simulink library "srx_platform"  (Simulink 8.2)
settings: Solver=ode1  StartTime=0.0  StopTime=Inf  FixedStep=0.001  RelTol=1e-3
PostLoadFcn:
  | , if any(exist('dsrtsu_mdlpostloadfcn', 'file') == [2, 3, 6]), try dsrtsu_mdlpostloadfcn('Execute', bdroot); catch fprintf('Error in PostLoadFcn (dsrtsu_mdlpostloadfcn) for model "%s":\n %s\n', bdroot, lasterr); end, end,
libraries: rtican x23, rtiethernetudplib x4, srx_initialize x4, rtiflashlib x2, topr5_adapter x1
(part 6 of 6)

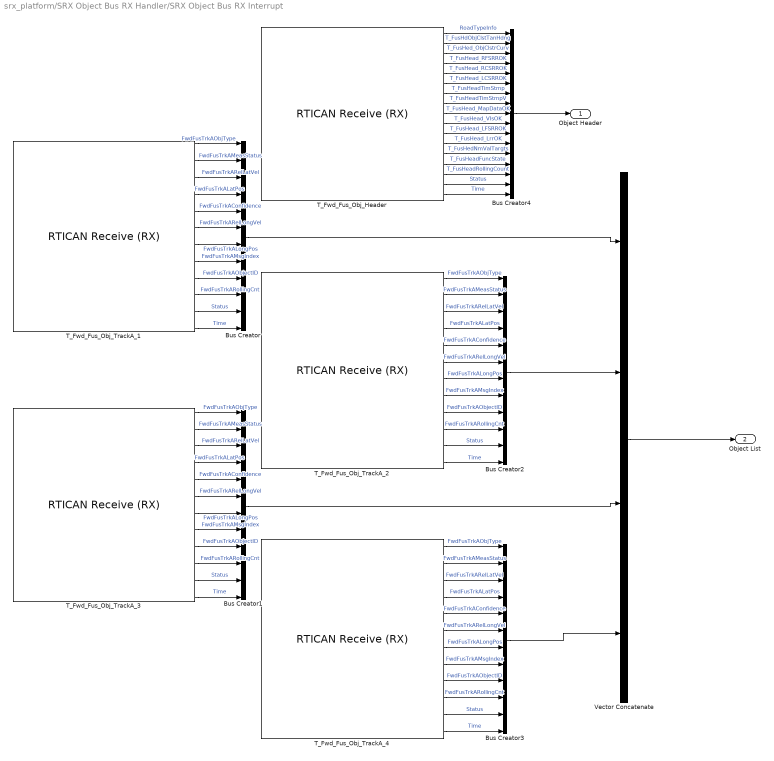
== system srx_platform/SRX Object Bus RX Handler/SRX Object Bus RX Interrupt ==
  Bus Creator{,1..3} (4 alike) : BusCreator  Inputs='FwdFusTrkAObjType','FwdFusTrkAMeasStatus','FwdFusTrkARelLatVel','FwdFusTrkALatPos','FwdFusTrkAConfidence','FwdFusTrkARelLongVel','FwdFusTrkALongPos','FwdFusTrkAMsgIndex','FwdFusTrkAObjectID','FwdFusTrkARollingCnt','Status','Time'  OutDataTypeStr=Bus: FusObjectTrackA  NonVirtualBus=on
  Bus Creator4 : BusCreator  Inputs=17
  T_Fwd_Fus_Obj_Header : rtican/RTICAN Receive (RX)   Reserved1=[]  Reserved2=[]  Reserved3=[]  Reserved4=[]  SfcnMessage=[]  Msg_Struct=[]  BoardTypeNo=[]  BoardNo=[]  ChannelNo=[]  Parameters=[]  DialogFcn=[]  UnitName=[]  Revision=[]  UnitValues=[]  DSProperties=struct('RTI',struct('Version',uint32(5),'BlockType',struct('isSLSource',uint8(1),'isSLSink',uint8(1),'isHWSource',uint8(0),'isHWSink',uint8(0),'isSetup',uint8(0),'isInline',uint8(1),'isNonInline',uint8(0),'isInterrupt',uint8(0),'isChannelwise',uint8(0)),'IOBoardType','RTICAN','UnitType','MESSAGE','Identifier','RX','DialogType','MSVC','BlockSet','RTICAN','SlaveProcessor','CAN'))  RTIBlockInterface=struct('OutputPortsWidth',int32([1 1 1 1 1 1 1 1 1 1 1 1 1 1 1 1 1]),'OutputPortsActive',[1 1 1 1 1 1 1 1 1 1 1 1 1 1 1 1 1],'OutputPortsName',{{'RoadTypeInfo','T_FusHdObjClstTanHdng','T_FusHed_ObjClstrCurv','T_FusHead_RFSRROK','T_FusHead_RCSRROK','T_FusHead_LCSRROK','T_FusHeadTimStmp','T_FusHeadTimStmpV','T_FusHead_MapDataOK','T_FusHead_VIsOK','T_FusHead_LFSRROK','T_FusHead_LrrOK','T_FusHedNmValTargts','T_FusHeadFuncState','T_FusHeadRollingCount',['RX status'],['RX time']}},'OutputPortsDataType',{{'SS_DOUBLE','SS_DOUBLE','SS_DOUBLE','SS_DOUBLE','SS_DOUBLE','SS_DOUBLE','SS_DOUBLE','SS_DOUBLE','SS_DOUBLE','SS_DOUBLE','SS_DOUBLE','SS_DOUBLE','SS_DOUBLE','SS_DOUBLE','SS_DOUBLE','SS_DOUBLE','SS_DOUBLE'}},'OutputPortsLabel',{{'RoadTypeInfo','T_FusHdObjClstTanHdng','T_FusHed_ObjClstrCurv','T_FusHead_RFSRROK','T_FusHead_RCSRROK','T_FusHead_LCSRROK','T_FusHeadTimStmp','T_FusHeadTimStmpV','T_FusHead_MapDataOK','T_FusHead_VIsOK','T_FusHead_LFSRROK','T_FusHead_LrrOK','T_FusHedNmValTargts','T_FusHeadFuncState','T_FusHeadRollingCount','',''}},'OutputPortsLabelMode','ON','InputPortsWidth',int32(0),'InputPortsActive',0,'DialogFcn','rtican_message_interface_gui','BlockDisplay',{{'','center'}},'IconTransparency','on','ParameterTunableNames',{{}},'InitLevel',3,'BlockName',struct('Token',{{'T_Fwd_Fus_Obj_Header'}}),'SampleTime',{{-1}},'TriggerPort',{{'none'}},'EnablePort',{{'none'}})  RTIBlockParameters=struct('BoardTypeNo',{{1,'OFF',[]}},'BoardNo',{{1,'ON',[1 16]}},'ChannelNo',{{2,'ON',[1 2]}},'Parameters',{{struct('DataFileSupport',struct('DataFileSelectedMaster',1,'DataFileSelectedLocal',0,'DataFileName','c:\users\leidos\development\carmaplatform\microautobox\src\data_files\globala_fo.dbc|','DataFileDate',{{{['23-Jul-2015 14:24:26']}}},'SelectedFile',['<no file selected>']),'Options',struct('StatusSelected',1,'TimeSelected',1,'DeltaTimeSelected',0,'BytePortSelected',0,'MessageLengthSelected',0,'TriggerPort',struct('Selected',0,'TriggerType',0),'UserCoding',struct('Selected',0,'InterfaceFile','UserDecodingFile','FcnName','UserDecodeFcn','InportSelected',0,'InportWidth',1,'OutportSelected',0,'OutportWidth',1),'EnablePortSelected',0,'SignalOnPortnameSelected',1,'UseRXService',1),'Message',struct('MsgOnBlocknameSelected',1,'MsgName','T_Fwd_Fus_Obj_Header','MsgIdFormat',0,'MsgId',1808,'MsgLength',7,'NumSignals',15,'SampleTime',-1,'Signal',struct('SgnName',{'RoadTypeInfo','T_FusHdObjClstTanHdng','T_FusHed_ObjClstrCurv','T_FusHead_RFSRROK','T_FusHead_RCSRROK','T_FusHead_LCSRROK','T_FusHeadTimStmp','T_FusHeadTimStmpV','T_FusHead_MapDataOK','T_FusHead_VIsOK','T_FusHead_LFSRROK','T_FusHead_LrrOK','T_FusHedNmValTargts','T_FusHeadFuncState','T_FusHeadRollingCount'},'SgnStartBit',{5,8,16,29,30,31,32,43,44,45,46,47,48,52,54},'SgnLength',{3,8,13,1,1,1,11,1,1,1,1,1,4,2,2},'SgnType',{0,0,0,0,0,0,0,0,0,0,0,0,0,0,0},'ModeValue',{-1,-1,-1,-1,-1,-1,-1,-1,-1,-1,-1,-1,-1,-1,-1},'DataType',{0,1,1,0,0,0,0,0,0,0,0,0,0,0,0},'ByteLayout',{2,2,2,2,2,2,2,2,2,2,2,2,2,2,2},'Factor',{1,0.002,5e-05,1,1,1,1,1,1,1,1,1,1,1,1},'Offset',{0,0,0,0,0,0,0,0,0,0,0,0,0,0,0},'SgnComment',{{''},{''},{''},{''},{''},{''},{''},{''},{''},{''},{''},{''},{''},{''},{''}},'SgnUnit',{'','m/m','1/m','','','','ms','','','','','','','',''},'Min',{0,-0.256,-0.2048,0,0,0,0,0,0,0,0,0,0,0,0},'Max',{7,0.254,0.20475,1,1,1,2047,1,1,1,1,1,15,3,3},'SLDataType',{'SS_DOUBLE','SS_DOUBLE','SS_DOUBLE','SS_DOUBLE','SS_DOUBLE','SS_DOUBLE','SS_DOUBLE','SS_DOUBLE','SS_DOUBLE','SS_DOUBLE','SS_DOUBLE','SS_DOUBLE','SS_DOUBLE','SS_DOUBLE','SS_DOUBLE'}),'MsgIdNumFormat',1,'MsgComment',{{''}}),'Version',1.2,'general',struct('isFromLib',0)),'OFF',[]}},'GroupId',{{struct('Group',{{'RTICAN'}},'No',2,'Behavior',{{'NAMECHANGE'}},'BlockType',{{'SINK'}},'NameChangeFlag',0),'OFF',[]}},'SFcnRTICANMessage',{{struct('MsgType','RX','SFcnPortType','Scalar','MsgName','T_Fwd_Fus_Obj_Header','MsgIdFormat','STD','MsgId',1808,'MsgLength',7,'NumSignals',15,'SampleTime',-1,'Signal',struct('SgnName',{'RoadTypeInfo','T_FusHdObjClstTanHdng','T_FusHed_ObjClstrCurv','T_FusHead_RFSRROK','T_FusHead_RCSRROK','T_FusHead_LCSRROK','T_FusHeadTimStmp','T_FusHeadTimStmpV','T_FusHead_MapDataOK','T_FusHead_VIsOK','T_FusHead_LFSRROK','T_FusHead_LrrOK','T_FusHedNmValTargts','T_FusHeadFuncState','T_FusHeadRollingCount'},'SgnStartBit',{5,8,16,29,30,31,32,43,44,45,46,47,48,52,54},'SgnLength',{3,8,13,1,1,1,11,1,1,1,1,1,4,2,2},'SgnType',{'standard','standard','standard','standard','standard','standard','standard','standard','standard','standard','standard','standard','standard','standard','standard'},'ModeValue',{-1,-1,-1,-1,-1,-1,-1,-1,-1,-1,-1,-1,-1,-1,-1},'DataType',{['unsigned int'],['signed int'],['signed int'],['unsigned int'],['unsigned int'],['unsigned int'],['unsigned int'],['unsigned int'],['unsigned int'],['unsigned int'],['unsigned int'],['unsigned int'],['unsigned int'],['unsigned int'],['unsigned int']},'ByteLayout',{['motorola back.'],['motorola back.'],['motorola back.'],['motorola back.'],['motorola back.'],['motorola back.'],['motorola back.'],['motorola back.'],['motorola back.'],['motorola back.'],['motorola back.'],['motorola back.'],['motorola back.'],['motorola back.'],['motorola back.']},'Factor',{1,0.002,5e-05,1,1,1,1,1,1,1,1,1,1,1,1},'Offset',{0,0,0,0,0,0,0,0,0,0,0,0,0,0,0},'SLDataType',{'SS_DOUBLE','SS_DOUBLE','SS_DOUBLE','SS_DOUBLE','SS_DOUBLE','SS_DOUBLE','SS_DOUBLE','SS_DOUBLE','SS_DOUBLE','SS_DOUBLE','SS_DOUBLE','SS_DOUBLE','SS_DOUBLE','SS_DOUBLE','SS_DOUBLE'}),'StatusSelected','yes','TimeSelected','yes','DeltaTimeSelected','no','BytePortSelected','no','MessageLengthSelected','no','TriggerPort',struct('Selected','no','TriggerType',0),'UserCoding',struct('Selected','no','InterfaceFile','UserDecodingFile','FcnName','UserDecodeFcn','InportSelected','no','InportWidth',1,'OutportSelected','no','OutportWidth',1),'EnablePortSelected','no','UseRXService','yes','BoardType','DS1','BoardNo',1,'ControllerNo',2),'OFF',[]}},'TLCFileName',{{'rtican_rx_message','OFF',[]}})  RTISFcnParameters=struct('SFcnRTICANMessage','struct','TLCFileName','char')  RTIBlockParaDefault=struct('BoardTypeNo',4302,'BoardNo',1,'ChannelNo',1,'Parameters',struct('DataFileSupport',struct('DataFileSelectedMaster',0,'DataFileSelectedLocal',0,'DataFileName','','DataFileDate','','SelectedFile',['<no file selected>']),'Options',struct('StatusSelected',1,'TimeSelected',1,'DeltaTimeSelected',1,'BytePortSelected',0,'MessageLengthSelected',0,'TriggerPort',struct('Selected',0,'TriggerType','rising'),'UserCoding',struct('Selected',0,'InterfaceFile','UserDecodingFile','FcnName','UserDecodeFcn','InportSelected',0,'InportWidth',1,'OutportSelected',0,'OutportWidth',1),'EnablePortSelected',0,'SignalOnPortnameSelected',1,'UseRXService',0),'Message',struct('MsgOnBlocknameSelected',0,'MsgName',['RX Message'],'MsgIdFormat',0,'MsgId',100,'MsgLength',8,'NumSignals',1,'SampleTime',-1,'Signal',struct('SgnName',['RX signal'],'SgnStartBit',0,'SgnLength',8,'SgnType',0,'ModeValue',-1,'DataType',0,'SLDataType','SS_DOUBLE','ByteLayout',0,'Factor',1,'Offset',0,'Min',0,'Max',255,'SgnComment',{{}},'SgnUnit',''),'MsgIdNumFormat',0,'MsgComment',{{''}}),'Version',1.2,'general',struct('isFromLib',1)),'GroupId',struct('Group',{{'RTICAN'}},'No',1,'Behavior',{{'NAMECHANGE'}},'BlockType',{{'SINK'}},'NameChangeFlag',0),'SFcnRTICANMessage',struct('MsgType','RX','MsgName',['RX Message'],'MsgIdFormat','STD','MsgId',100,'MsgLength',8,'NumSignals',1,'SampleTime',-1,'Signal',struct('SgnName',['RX signal'],'SgnStartBit',0,'SgnLength',8,'SgnType','standard','ModeValue',-1,'DataType',['unsigned int'],'ByteLayout',['little endian'],'SLDataType','SS_DOUBLE','Factor',1,'Offset',0),'StatusSelected','yes','TimeSelected','yes','DeltaTimeSelected','yes','BytePortSelected','no','MessageLengthSelected','no','EnablePortSelected','no','UserCoding',struct('Selected','no','InterfaceFile','UserDecodingFile','FcnName','UserDecodeFcn','InportSelected','no','InportWidth',1,'OutportSelected','no','OutportWidth',1),'TriggerPort',struct('Selected','no','TriggerType','rising'),'UseRXService','no','BoardType','DS4302','BoardNo',1,'ControllerNo',1,'SFcnPortType','Scalar'),'TLCFileName','rtican_rx_message')
      settings: AttributesFormatString=Group Id: RTICAN2\n
  T_Fwd_Fus_Obj_TrackA_1 : rtican/RTICAN Receive (RX)   Reserved1=[]  Reserved2=[]  Reserved3=[]  Reserved4=[]  SfcnMessage=[]  Msg_Struct=[]  BoardTypeNo=[]  BoardNo=[]  ChannelNo=[]  Parameters=[]  DialogFcn=[]  UnitName=[]  Revision=[]  UnitValues=[]  DSProperties=struct('RTI',struct('Version',uint32(5),'BlockType',struct('isSLSource',uint8(1),'isSLSink',uint8(1),'isHWSource',uint8(0),'isHWSink',uint8(0),'isSetup',uint8(0),'isInline',uint8(1),'isNonInline',uint8(0),'isInterrupt',uint8(0),'isChannelwise',uint8(0)),'IOBoardType','RTICAN','UnitType','MESSAGE','Identifier','RX','DialogType','MSVC','BlockSet','RTICAN','SlaveProcessor','CAN'))  RTIBlockInterface=struct('OutputPortsWidth',int32([1 1 1 1 1 1 1 1 1 1 1 1]),'OutputPortsActive',[1 1 1 1 1 1 1 1 1 1 1 1],'OutputPortsName',{{'FwdFusTrkAObjType','FwdFusTrkAMeasStatus','FwdFusTrkARelLatVel','FwdFusTrkALatPos','FwdFusTrkAConfidence','FwdFusTrkARelLongVel','FwdFusTrkALongPos','FwdFusTrkAMsgIndex','FwdFusTrkAObjectID','FwdFusTrkARollingCnt',['RX status'],['RX time']}},'OutputPortsDataType',{{'SS_DOUBLE','SS_DOUBLE','SS_DOUBLE','SS_DOUBLE','SS_DOUBLE','SS_DOUBLE','SS_DOUBLE','SS_DOUBLE','SS_DOUBLE','SS_DOUBLE','SS_DOUBLE','SS_DOUBLE'}},'OutputPortsLabel',{{'FwdFusTrkAObjType','FwdFusTrkAMeasStatus','FwdFusTrkARelLatVel','FwdFusTrkALatPos','FwdFusTrkAConfidence','FwdFusTrkARelLongVel','FwdFusTrkALongPos','FwdFusTrkAMsgIndex','FwdFusTrkAObjectID','FwdFusTrkARollingCnt','',''}},'OutputPortsLabelMode','ON','InputPortsWidth',int32(0),'InputPortsActive',0,'DialogFcn','rtican_message_interface_gui','BlockDisplay',{{'','center'}},'IconTransparency','on','ParameterTunableNames',{{}},'InitLevel',3,'BlockName',struct('Token',{{'T_Fwd_Fus_Obj_TrackA_1'}}),'SampleTime',{{-1}},'TriggerPort',{{'none'}},'EnablePort',{{'none'}})  RTIBlockParameters=struct('BoardTypeNo',{{1,'OFF',[]}},'BoardNo',{{1,'ON',[1 16]}},'ChannelNo',{{2,'ON',[1 2]}},'Parameters',{{struct('DataFileSupport',struct('DataFileSelectedMaster',1,'DataFileSelectedLocal',0,'DataFileName','c:\users\leidos\development\carmaplatform\microautobox\src\data_files\globala_fo.dbc|','DataFileDate',{{{['23-Jul-2015 14:24:26']}}},'SelectedFile',['<no file selected>']),'Options',struct('StatusSelected',1,'TimeSelected',1,'DeltaTimeSelected',0,'BytePortSelected',0,'MessageLengthSelected',0,'TriggerPort',struct('Selected',0,'TriggerType',0),'UserCoding',struct('Selected',0,'InterfaceFile','UserDecodingFile','FcnName','UserDecodeFcn','InportSelected',0,'InportWidth',1,'OutportSelected',0,'OutportWidth',1),'EnablePortSelected',0,'SignalOnPortnameSelected',1,'UseRXService',1),'Message',struct('MsgOnBlocknameSelected',1,'MsgName','T_Fwd_Fus_Obj_TrackA_1','MsgIdFormat',0,'MsgId',1809,'MsgLength',8,'NumSignals',10,'SampleTime',-1,'Signal',struct('SgnName',{'FwdFusTrkAObjType','FwdFusTrkAMeasStatus','FwdFusTrkARelLatVel','FwdFusTrkALatPos','FwdFusTrkAConfidence','FwdFusTrkARelLongVel','FwdFusTrkALongPos','FwdFusTrkAMsgIndex','FwdFusTrkAObjectID','FwdFusTrkARollingCnt'},'SgnStartBit',{0,3,5,16,27,29,40,52,56,62},'SgnLength',{3,2,11,11,2,11,12,4,6,2},'SgnType',{0,0,0,0,0,0,0,0,0,0},'ModeValue',{-1,-1,-1,-1,-1,-1,-1,-1,-1,-1},'DataType',{0,0,1,1,0,1,1,0,0,0},'ByteLayout',{2,2,2,2,2,2,2,2,2,2},'Factor',{1,1,0.125,0.125,1,0.125,0.125,1,1,1},'Offset',{0,0,0,0,0,0,0,0,0,0},'SgnComment',{{''},{''},{''},{''},{''},{''},{''},{''},{''},{''}},'SgnUnit',{'','','m/s','m','','m/s','m','','',''},'Min',{0,0,-128,-128,0,-128,-256,0,0,0},'Max',{7,3,127.875,127.875,3,127.875,255.875,15,63,3},'SLDataType',{'SS_DOUBLE','SS_DOUBLE','SS_DOUBLE','SS_DOUBLE','SS_DOUBLE','SS_DOUBLE','SS_DOUBLE','SS_DOUBLE','SS_DOUBLE','SS_DOUBLE'}),'MsgIdNumFormat',1,'MsgComment',{{''}}),'Version',1.2,'general',struct('isFromLib',0)),'OFF',[]}},'GroupId',{{struct('Group',{{'RTICAN'}},'No',2,'Behavior',{{'NAMECHANGE'}},'BlockType',{{'SINK'}},'NameChangeFlag',0),'OFF',[]}},'SFcnRTICANMessage',{{struct('MsgType','RX','SFcnPortType','Scalar','MsgName','T_Fwd_Fus_Obj_TrackA_1','MsgIdFormat','STD','MsgId',1809,'MsgLength',8,'NumSignals',10,'SampleTime',-1,'Signal',struct('SgnName',{'FwdFusTrkAObjType','FwdFusTrkAMeasStatus','FwdFusTrkARelLatVel','FwdFusTrkALatPos','FwdFusTrkAConfidence','FwdFusTrkARelLongVel','FwdFusTrkALongPos','FwdFusTrkAMsgIndex','FwdFusTrkAObjectID','FwdFusTrkARollingCnt'},'SgnStartBit',{0,3,5,16,27,29,40,52,56,62},'SgnLength',{3,2,11,11,2,11,12,4,6,2},'SgnType',{'standard','standard','standard','standard','standard','standard','standard','standard','standard','standard'},'ModeValue',{-1,-1,-1,-1,-1,-1,-1,-1,-1,-1},'DataType',{['unsigned int'],['unsigned int'],['signed int'],['signed int'],['unsigned int'],['signed int'],['signed int'],['unsigned int'],['unsigned int'],['unsigned int']},'ByteLayout',{['motorola back.'],['motorola back.'],['motorola back.'],['motorola back.'],['motorola back.'],['motorola back.'],['motorola back.'],['motorola back.'],['motorola back.'],['motorola back.']},'Factor',{1,1,0.125,0.125,1,0.125,0.125,1,1,1},'Offset',{0,0,0,0,0,0,0,0,0,0},'SLDataType',{'SS_DOUBLE','SS_DOUBLE','SS_DOUBLE','SS_DOUBLE','SS_DOUBLE','SS_DOUBLE','SS_DOUBLE','SS_DOUBLE','SS_DOUBLE','SS_DOUBLE'}),'StatusSelected','yes','TimeSelected','yes','DeltaTimeSelected','no','BytePortSelected','no','MessageLengthSelected','no','TriggerPort',struct('Selected','no','TriggerType',0),'UserCoding',struct('Selected','no','InterfaceFile','UserDecodingFile','FcnName','UserDecodeFcn','InportSelected','no','InportWidth',1,'OutportSelected','no','OutportWidth',1),'EnablePortSelected','no','UseRXService','yes','BoardType','DS1','BoardNo',1,'ControllerNo',2),'OFF',[]}},'TLCFileName',{{'rtican_rx_message','OFF',[]}})  RTISFcnParameters=struct('SFcnRTICANMessage','struct','TLCFileName','char')  RTIBlockParaDefault=struct('BoardTypeNo',4302,'BoardNo',1,'ChannelNo',1,'Parameters',struct('DataFileSupport',struct('DataFileSelectedMaster',0,'DataFileSelectedLocal',0,'DataFileName','','DataFileDate','','SelectedFile',['<no file selected>']),'Options',struct('StatusSelected',1,'TimeSelected',1,'DeltaTimeSelected',1,'BytePortSelected',0,'MessageLengthSelected',0,'TriggerPort',struct('Selected',0,'TriggerType','rising'),'UserCoding',struct('Selected',0,'InterfaceFile','UserDecodingFile','FcnName','UserDecodeFcn','InportSelected',0,'InportWidth',1,'OutportSelected',0,'OutportWidth',1),'EnablePortSelected',0,'SignalOnPortnameSelected',1,'UseRXService',0),'Message',struct('MsgOnBlocknameSelected',0,'MsgName',['RX Message'],'MsgIdFormat',0,'MsgId',100,'MsgLength',8,'NumSignals',1,'SampleTime',-1,'Signal',struct('SgnName',['RX signal'],'SgnStartBit',0,'SgnLength',8,'SgnType',0,'ModeValue',-1,'DataType',0,'SLDataType','SS_DOUBLE','ByteLayout',0,'Factor',1,'Offset',0,'Min',0,'Max',255,'SgnComment',{{}},'SgnUnit',''),'MsgIdNumFormat',0,'MsgComment',{{''}}),'Version',1.2,'general',struct('isFromLib',1)),'GroupId',struct('Group',{{'RTICAN'}},'No',1,'Behavior',{{'NAMECHANGE'}},'BlockType',{{'SINK'}},'NameChangeFlag',0),'SFcnRTICANMessage',struct('MsgType','RX','MsgName',['RX Message'],'MsgIdFormat','STD','MsgId',100,'MsgLength',8,'NumSignals',1,'SampleTime',-1,'Signal',struct('SgnName',['RX signal'],'SgnStartBit',0,'SgnLength',8,'SgnType','standard','ModeValue',-1,'DataType',['unsigned int'],'ByteLayout',['little endian'],'SLDataType','SS_DOUBLE','Factor',1,'Offset',0),'StatusSelected','yes','TimeSelected','yes','DeltaTimeSelected','yes','BytePortSelected','no','MessageLengthSelected','no','EnablePortSelected','no','UserCoding',struct('Selected','no','InterfaceFile','UserDecodingFile','FcnName','UserDecodeFcn','InportSelected','no','InportWidth',1,'OutportSelected','no','OutportWidth',1),'TriggerPort',struct('Selected','no','TriggerType','rising'),'UseRXService','no','BoardType','DS4302','BoardNo',1,'ControllerNo',1,'SFcnPortType','Scalar'),'TLCFileName','rtican_rx_message')
      settings: AttributesFormatString=Group Id: RTICAN2\n
  T_Fwd_Fus_Obj_TrackA_2 : rtican/RTICAN Receive (RX)   Reserved1=[]  Reserved2=[]  Reserved3=[]  Reserved4=[]  SfcnMessage=[]  Msg_Struct=[]  BoardTypeNo=[]  BoardNo=[]  ChannelNo=[]  Parameters=[]  DialogFcn=[]  UnitName=[]  Revision=[]  UnitValues=[]  DSProperties=struct('RTI',struct('Version',uint32(5),'BlockType',struct('isSLSource',uint8(1),'isSLSink',uint8(1),'isHWSource',uint8(0),'isHWSink',uint8(0),'isSetup',uint8(0),'isInline',uint8(1),'isNonInline',uint8(0),'isInterrupt',uint8(0),'isChannelwise',uint8(0)),'IOBoardType','RTICAN','UnitType','MESSAGE','Identifier','RX','DialogType','MSVC','BlockSet','RTICAN','SlaveProcessor','CAN'))  RTIBlockInterface=struct('OutputPortsWidth',int32([1 1 1 1 1 1 1 1 1 1 1 1]),'OutputPortsActive',[1 1 1 1 1 1 1 1 1 1 1 1],'OutputPortsName',{{'FwdFusTrkAObjType','FwdFusTrkAMeasStatus','FwdFusTrkARelLatVel','FwdFusTrkALatPos','FwdFusTrkAConfidence','FwdFusTrkARelLongVel','FwdFusTrkALongPos','FwdFusTrkAMsgIndex','FwdFusTrkAObjectID','FwdFusTrkARollingCnt',['RX status'],['RX time']}},'OutputPortsDataType',{{'SS_DOUBLE','SS_DOUBLE','SS_DOUBLE','SS_DOUBLE','SS_DOUBLE','SS_DOUBLE','SS_DOUBLE','SS_DOUBLE','SS_DOUBLE','SS_DOUBLE','SS_DOUBLE','SS_DOUBLE'}},'OutputPortsLabel',{{'FwdFusTrkAObjType','FwdFusTrkAMeasStatus','FwdFusTrkARelLatVel','FwdFusTrkALatPos','FwdFusTrkAConfidence','FwdFusTrkARelLongVel','FwdFusTrkALongPos','FwdFusTrkAMsgIndex','FwdFusTrkAObjectID','FwdFusTrkARollingCnt','',''}},'OutputPortsLabelMode','ON','InputPortsWidth',int32(0),'InputPortsActive',0,'DialogFcn','rtican_message_interface_gui','BlockDisplay',{{'','center'}},'IconTransparency','on','ParameterTunableNames',{{}},'InitLevel',3,'BlockName',struct('Token',{{'T_Fwd_Fus_Obj_TrackA_1'}}),'SampleTime',{{-1}},'TriggerPort',{{'none'}},'EnablePort',{{'none'}})  RTIBlockParameters=struct('BoardTypeNo',{{1,'OFF',[]}},'BoardNo',{{1,'ON',[1 16]}},'ChannelNo',{{2,'ON',[1 2]}},'Parameters',{{struct('DataFileSupport',struct('DataFileSelectedMaster',1,'DataFileSelectedLocal',0,'DataFileName','c:\users\leidos\development\carmaplatform\microautobox\src\data_files\globala_fo.dbc|','DataFileDate',{{{['23-Jul-2015 14:24:26']}}},'SelectedFile',['<no file selected>']),'Options',struct('StatusSelected',1,'TimeSelected',1,'DeltaTimeSelected',0,'BytePortSelected',0,'MessageLengthSelected',0,'TriggerPort',struct('Selected',0,'TriggerType',0),'UserCoding',struct('Selected',0,'InterfaceFile','UserDecodingFile','FcnName','UserDecodeFcn','InportSelected',0,'InportWidth',1,'OutportSelected',0,'OutportWidth',1),'EnablePortSelected',0,'SignalOnPortnameSelected',1,'UseRXService',1),'Message',struct('MsgOnBlocknameSelected',1,'MsgName','T_Fwd_Fus_Obj_TrackA_2','MsgIdFormat',0,'MsgId',1810,'MsgLength',8,'NumSignals',10,'SampleTime',-1,'Signal',struct('SgnName',{'FwdFusTrkAObjType','FwdFusTrkAMeasStatus','FwdFusTrkARelLatVel','FwdFusTrkALatPos','FwdFusTrkAConfidence','FwdFusTrkARelLongVel','FwdFusTrkALongPos','FwdFusTrkAMsgIndex','FwdFusTrkAObjectID','FwdFusTrkARollingCnt'},'SgnStartBit',{0,3,5,16,27,29,40,52,56,62},'SgnLength',{3,2,11,11,2,11,12,4,6,2},'SgnType',{0,0,0,0,0,0,0,0,0,0},'ModeValue',{-1,-1,-1,-1,-1,-1,-1,-1,-1,-1},'DataType',{0,0,1,1,0,1,1,0,0,0},'ByteLayout',{2,2,2,2,2,2,2,2,2,2},'Factor',{1,1,0.125,0.125,1,0.125,0.125,1,1,1},'Offset',{0,0,0,0,0,0,0,0,0,0},'SgnComment',{{''},{''},{''},{''},{''},{''},{''},{''},{''},{''}},'SgnUnit',{'','','m/s','m','','m/s','m','','',''},'Min',{0,0,-128,-128,0,-128,-256,0,0,0},'Max',{7,3,127.875,127.875,3,127.875,255.875,15,63,3},'SLDataType',{'SS_DOUBLE','SS_DOUBLE','SS_DOUBLE','SS_DOUBLE','SS_DOUBLE','SS_DOUBLE','SS_DOUBLE','SS_DOUBLE','SS_DOUBLE','SS_DOUBLE'}),'MsgIdNumFormat',1,'MsgComment',{{''}}),'Version',1.2,'general',struct('isFromLib',0)),'OFF',[]}},'GroupId',{{struct('Group',{{'RTICAN'}},'No',2,'Behavior',{{'NAMECHANGE'}},'BlockType',{{'SINK'}},'NameChangeFlag',0),'OFF',[]}},'SFcnRTICANMessage',{{struct('MsgType','RX','SFcnPortType','Scalar','MsgName','T_Fwd_Fus_Obj_TrackA_2','MsgIdFormat','STD','MsgId',1810,'MsgLength',8,'NumSignals',10,'SampleTime',-1,'Signal',struct('SgnName',{'FwdFusTrkAObjType','FwdFusTrkAMeasStatus','FwdFusTrkARelLatVel','FwdFusTrkALatPos','FwdFusTrkAConfidence','FwdFusTrkARelLongVel','FwdFusTrkALongPos','FwdFusTrkAMsgIndex','FwdFusTrkAObjectID','FwdFusTrkARollingCnt'},'SgnStartBit',{0,3,5,16,27,29,40,52,56,62},'SgnLength',{3,2,11,11,2,11,12,4,6,2},'SgnType',{'standard','standard','standard','standard','standard','standard','standard','standard','standard','standard'},'ModeValue',{-1,-1,-1,-1,-1,-1,-1,-1,-1,-1},'DataType',{['unsigned int'],['unsigned int'],['signed int'],['signed int'],['unsigned int'],['signed int'],['signed int'],['unsigned int'],['unsigned int'],['unsigned int']},'ByteLayout',{['motorola back.'],['motorola back.'],['motorola back.'],['motorola back.'],['motorola back.'],['motorola back.'],['motorola back.'],['motorola back.'],['motorola back.'],['motorola back.']},'Factor',{1,1,0.125,0.125,1,0.125,0.125,1,1,1},'Offset',{0,0,0,0,0,0,0,0,0,0},'SLDataType',{'SS_DOUBLE','SS_DOUBLE','SS_DOUBLE','SS_DOUBLE','SS_DOUBLE','SS_DOUBLE','SS_DOUBLE','SS_DOUBLE','SS_DOUBLE','SS_DOUBLE'}),'StatusSelected','yes','TimeSelected','yes','DeltaTimeSelected','no','BytePortSelected','no','MessageLengthSelected','no','TriggerPort',struct('Selected','no','TriggerType',0),'UserCoding',struct('Selected','no','InterfaceFile','UserDecodingFile','FcnName','UserDecodeFcn','InportSelected','no','InportWidth',1,'OutportSelected','no','OutportWidth',1),'EnablePortSelected','no','UseRXService','yes','BoardType','DS1','BoardNo',1,'ControllerNo',2),'OFF',[]}},'TLCFileName',{{'rtican_rx_message','OFF',[]}})  RTISFcnParameters=struct('SFcnRTICANMessage','struct','TLCFileName','char')  RTIBlockParaDefault=struct('BoardTypeNo',4302,'BoardNo',1,'ChannelNo',1,'Parameters',struct('DataFileSupport',struct('DataFileSelectedMaster',0,'DataFileSelectedLocal',0,'DataFileName','','DataFileDate','','SelectedFile',['<no file selected>']),'Options',struct('StatusSelected',1,'TimeSelected',1,'DeltaTimeSelected',1,'BytePortSelected',0,'MessageLengthSelected',0,'TriggerPort',struct('Selected',0,'TriggerType','rising'),'UserCoding',struct('Selected',0,'InterfaceFile','UserDecodingFile','FcnName','UserDecodeFcn','InportSelected',0,'InportWidth',1,'OutportSelected',0,'OutportWidth',1),'EnablePortSelected',0,'SignalOnPortnameSelected',1,'UseRXService',0),'Message',struct('MsgOnBlocknameSelected',0,'MsgName',['RX Message'],'MsgIdFormat',0,'MsgId',100,'MsgLength',8,'NumSignals',1,'SampleTime',-1,'Signal',struct('SgnName',['RX signal'],'SgnStartBit',0,'SgnLength',8,'SgnType',0,'ModeValue',-1,'DataType',0,'SLDataType','SS_DOUBLE','ByteLayout',0,'Factor',1,'Offset',0,'Min',0,'Max',255,'SgnComment',{{}},'SgnUnit',''),'MsgIdNumFormat',0,'MsgComment',{{''}}),'Version',1.2,'general',struct('isFromLib',1)),'GroupId',struct('Group',{{'RTICAN'}},'No',1,'Behavior',{{'NAMECHANGE'}},'BlockType',{{'SINK'}},'NameChangeFlag',0),'SFcnRTICANMessage',struct('MsgType','RX','MsgName',['RX Message'],'MsgIdFormat','STD','MsgId',100,'MsgLength',8,'NumSignals',1,'SampleTime',-1,'Signal',struct('SgnName',['RX signal'],'SgnStartBit',0,'SgnLength',8,'SgnType','standard','ModeValue',-1,'DataType',['unsigned int'],'ByteLayout',['little endian'],'SLDataType','SS_DOUBLE','Factor',1,'Offset',0),'StatusSelected','yes','TimeSelected','yes','DeltaTimeSelected','yes','BytePortSelected','no','MessageLengthSelected','no','EnablePortSelected','no','UserCoding',struct('Selected','no','InterfaceFile','UserDecodingFile','FcnName','UserDecodeFcn','InportSelected','no','InportWidth',1,'OutportSelected','no','OutportWidth',1),'TriggerPort',struct('Selected','no','TriggerType','rising'),'UseRXService','no','BoardType','DS4302','BoardNo',1,'ControllerNo',1,'SFcnPortType','Scalar'),'TLCFileName','rtican_rx_message')
      settings: AttributesFormatString=Group Id: RTICAN2\n
  T_Fwd_Fus_Obj_TrackA_3 : rtican/RTICAN Receive (RX)   Reserved1=[]  Reserved2=[]  Reserved3=[]  Reserved4=[]  SfcnMessage=[]  Msg_Struct=[]  BoardTypeNo=[]  BoardNo=[]  ChannelNo=[]  Parameters=[]  DialogFcn=[]  UnitName=[]  Revision=[]  UnitValues=[]  DSProperties=struct('RTI',struct('Version',uint32(5),'BlockType',struct('isSLSource',uint8(1),'isSLSink',uint8(1),'isHWSource',uint8(0),'isHWSink',uint8(0),'isSetup',uint8(0),'isInline',uint8(1),'isNonInline',uint8(0),'isInterrupt',uint8(0),'isChannelwise',uint8(0)),'IOBoardType','RTICAN','UnitType','MESSAGE','Identifier','RX','DialogType','MSVC','BlockSet','RTICAN','SlaveProcessor','CAN'))  RTIBlockInterface=struct('OutputPortsWidth',int32([1 1 1 1 1 1 1 1 1 1 1 1]),'OutputPortsActive',[1 1 1 1 1 1 1 1 1 1 1 1],'OutputPortsName',{{'FwdFusTrkAObjType','FwdFusTrkAMeasStatus','FwdFusTrkARelLatVel','FwdFusTrkALatPos','FwdFusTrkAConfidence','FwdFusTrkARelLongVel','FwdFusTrkALongPos','FwdFusTrkAMsgIndex','FwdFusTrkAObjectID','FwdFusTrkARollingCnt',['RX status'],['RX time']}},'OutputPortsDataType',{{'SS_DOUBLE','SS_DOUBLE','SS_DOUBLE','SS_DOUBLE','SS_DOUBLE','SS_DOUBLE','SS_DOUBLE','SS_DOUBLE','SS_DOUBLE','SS_DOUBLE','SS_DOUBLE','SS_DOUBLE'}},'OutputPortsLabel',{{'FwdFusTrkAObjType','FwdFusTrkAMeasStatus','FwdFusTrkARelLatVel','FwdFusTrkALatPos','FwdFusTrkAConfidence','FwdFusTrkARelLongVel','FwdFusTrkALongPos','FwdFusTrkAMsgIndex','FwdFusTrkAObjectID','FwdFusTrkARollingCnt','',''}},'OutputPortsLabelMode','ON','InputPortsWidth',int32(0),'InputPortsActive',0,'DialogFcn','rtican_message_interface_gui','BlockDisplay',{{'','center'}},'IconTransparency','on','ParameterTunableNames',{{}},'InitLevel',3,'BlockName',struct('Token',{{'T_Fwd_Fus_Obj_TrackA_1'}}),'SampleTime',{{-1}},'TriggerPort',{{'none'}},'EnablePort',{{'none'}})  RTIBlockParameters=struct('BoardTypeNo',{{1,'OFF',[]}},'BoardNo',{{1,'ON',[1 16]}},'ChannelNo',{{2,'ON',[1 2]}},'Parameters',{{struct('DataFileSupport',struct('DataFileSelectedMaster',1,'DataFileSelectedLocal',0,'DataFileName','c:\users\leidos\development\carmaplatform\microautobox\src\data_files\globala_fo.dbc|','DataFileDate',{{{['23-Jul-2015 14:24:26']}}},'SelectedFile',['<no file selected>']),'Options',struct('StatusSelected',1,'TimeSelected',1,'DeltaTimeSelected',0,'BytePortSelected',0,'MessageLengthSelected',0,'TriggerPort',struct('Selected',0,'TriggerType',0),'UserCoding',struct('Selected',0,'InterfaceFile','UserDecodingFile','FcnName','UserDecodeFcn','InportSelected',0,'InportWidth',1,'OutportSelected',0,'OutportWidth',1),'EnablePortSelected',0,'SignalOnPortnameSelected',1,'UseRXService',1),'Message',struct('MsgOnBlocknameSelected',1,'MsgName','T_Fwd_Fus_Obj_TrackA_3','MsgIdFormat',0,'MsgId',1811,'MsgLength',8,'NumSignals',10,'SampleTime',-1,'Signal',struct('SgnName',{'FwdFusTrkAObjType','FwdFusTrkAMeasStatus','FwdFusTrkARelLatVel','FwdFusTrkALatPos','FwdFusTrkAConfidence','FwdFusTrkARelLongVel','FwdFusTrkALongPos','FwdFusTrkAMsgIndex','FwdFusTrkAObjectID','FwdFusTrkARollingCnt'},'SgnStartBit',{0,3,5,16,27,29,40,52,56,62},'SgnLength',{3,2,11,11,2,11,12,4,6,2},'SgnType',{0,0,0,0,0,0,0,0,0,0},'ModeValue',{-1,-1,-1,-1,-1,-1,-1,-1,-1,-1},'DataType',{0,0,1,1,0,1,1,0,0,0},'ByteLayout',{2,2,2,2,2,2,2,2,2,2},'Factor',{1,1,0.125,0.125,1,0.125,0.125,1,1,1},'Offset',{0,0,0,0,0,0,0,0,0,0},'SgnComment',{{''},{''},{''},{''},{''},{''},{''},{''},{''},{''}},'SgnUnit',{'','','m/s','m','','m/s','m','','',''},'Min',{0,0,-128,-128,0,-128,-256,0,0,0},'Max',{7,3,127.875,127.875,3,127.875,255.875,15,63,3},'SLDataType',{'SS_DOUBLE','SS_DOUBLE','SS_DOUBLE','SS_DOUBLE','SS_DOUBLE','SS_DOUBLE','SS_DOUBLE','SS_DOUBLE','SS_DOUBLE','SS_DOUBLE'}),'MsgIdNumFormat',1,'MsgComment',{{''}}),'Version',1.2,'general',struct('isFromLib',0)),'OFF',[]}},'GroupId',{{struct('Group',{{'RTICAN'}},'No',2,'Behavior',{{'NAMECHANGE'}},'BlockType',{{'SINK'}},'NameChangeFlag',0),'OFF',[]}},'SFcnRTICANMessage',{{struct('MsgType','RX','SFcnPortType','Scalar','MsgName','T_Fwd_Fus_Obj_TrackA_3','MsgIdFormat','STD','MsgId',1811,'MsgLength',8,'NumSignals',10,'SampleTime',-1,'Signal',struct('SgnName',{'FwdFusTrkAObjType','FwdFusTrkAMeasStatus','FwdFusTrkARelLatVel','FwdFusTrkALatPos','FwdFusTrkAConfidence','FwdFusTrkARelLongVel','FwdFusTrkALongPos','FwdFusTrkAMsgIndex','FwdFusTrkAObjectID','FwdFusTrkARollingCnt'},'SgnStartBit',{0,3,5,16,27,29,40,52,56,62},'SgnLength',{3,2,11,11,2,11,12,4,6,2},'SgnType',{'standard','standard','standard','standard','standard','standard','standard','standard','standard','standard'},'ModeValue',{-1,-1,-1,-1,-1,-1,-1,-1,-1,-1},'DataType',{['unsigned int'],['unsigned int'],['signed int'],['signed int'],['unsigned int'],['signed int'],['signed int'],['unsigned int'],['unsigned int'],['unsigned int']},'ByteLayout',{['motorola back.'],['motorola back.'],['motorola back.'],['motorola back.'],['motorola back.'],['motorola back.'],['motorola back.'],['motorola back.'],['motorola back.'],['motorola back.']},'Factor',{1,1,0.125,0.125,1,0.125,0.125,1,1,1},'Offset',{0,0,0,0,0,0,0,0,0,0},'SLDataType',{'SS_DOUBLE','SS_DOUBLE','SS_DOUBLE','SS_DOUBLE','SS_DOUBLE','SS_DOUBLE','SS_DOUBLE','SS_DOUBLE','SS_DOUBLE','SS_DOUBLE'}),'StatusSelected','yes','TimeSelected','yes','DeltaTimeSelected','no','BytePortSelected','no','MessageLengthSelected','no','TriggerPort',struct('Selected','no','TriggerType',0),'UserCoding',struct('Selected','no','InterfaceFile','UserDecodingFile','FcnName','UserDecodeFcn','InportSelected','no','InportWidth',1,'OutportSelected','no','OutportWidth',1),'EnablePortSelected','no','UseRXService','yes','BoardType','DS1','BoardNo',1,'ControllerNo',2),'OFF',[]}},'TLCFileName',{{'rtican_rx_message','OFF',[]}})  RTISFcnParameters=struct('SFcnRTICANMessage','struct','TLCFileName','char')  RTIBlockParaDefault=struct('BoardTypeNo',4302,'BoardNo',1,'ChannelNo',1,'Parameters',struct('DataFileSupport',struct('DataFileSelectedMaster',0,'DataFileSelectedLocal',0,'DataFileName','','DataFileDate','','SelectedFile',['<no file selected>']),'Options',struct('StatusSelected',1,'TimeSelected',1,'DeltaTimeSelected',1,'BytePortSelected',0,'MessageLengthSelected',0,'TriggerPort',struct('Selected',0,'TriggerType','rising'),'UserCoding',struct('Selected',0,'InterfaceFile','UserDecodingFile','FcnName','UserDecodeFcn','InportSelected',0,'InportWidth',1,'OutportSelected',0,'OutportWidth',1),'EnablePortSelected',0,'SignalOnPortnameSelected',1,'UseRXService',0),'Message',struct('MsgOnBlocknameSelected',0,'MsgName',['RX Message'],'MsgIdFormat',0,'MsgId',100,'MsgLength',8,'NumSignals',1,'SampleTime',-1,'Signal',struct('SgnName',['RX signal'],'SgnStartBit',0,'SgnLength',8,'SgnType',0,'ModeValue',-1,'DataType',0,'SLDataType','SS_DOUBLE','ByteLayout',0,'Factor',1,'Offset',0,'Min',0,'Max',255,'SgnComment',{{}},'SgnUnit',''),'MsgIdNumFormat',0,'MsgComment',{{''}}),'Version',1.2,'general',struct('isFromLib',1)),'GroupId',struct('Group',{{'RTICAN'}},'No',1,'Behavior',{{'NAMECHANGE'}},'BlockType',{{'SINK'}},'NameChangeFlag',0),'SFcnRTICANMessage',struct('MsgType','RX','MsgName',['RX Message'],'MsgIdFormat','STD','MsgId',100,'MsgLength',8,'NumSignals',1,'SampleTime',-1,'Signal',struct('SgnName',['RX signal'],'SgnStartBit',0,'SgnLength',8,'SgnType','standard','ModeValue',-1,'DataType',['unsigned int'],'ByteLayout',['little endian'],'SLDataType','SS_DOUBLE','Factor',1,'Offset',0),'StatusSelected','yes','TimeSelected','yes','DeltaTimeSelected','yes','BytePortSelected','no','MessageLengthSelected','no','EnablePortSelected','no','UserCoding',struct('Selected','no','InterfaceFile','UserDecodingFile','FcnName','UserDecodeFcn','InportSelected','no','InportWidth',1,'OutportSelected','no','OutportWidth',1),'TriggerPort',struct('Selected','no','TriggerType','rising'),'UseRXService','no','BoardType','DS4302','BoardNo',1,'ControllerNo',1,'SFcnPortType','Scalar'),'TLCFileName','rtican_rx_message')
      settings: AttributesFormatString=Group Id: RTICAN2\n
  T_Fwd_Fus_Obj_TrackA_4 : rtican/RTICAN Receive (RX)   Reserved1=[]  Reserved2=[]  Reserved3=[]  Reserved4=[]  SfcnMessage=[]  Msg_Struct=[]  BoardTypeNo=[]  BoardNo=[]  ChannelNo=[]  Parameters=[]  DialogFcn=[]  UnitName=[]  Revision=[]  UnitValues=[]  DSProperties=struct('RTI',struct('Version',uint32(5),'BlockType',struct('isSLSource',uint8(1),'isSLSink',uint8(1),'isHWSource',uint8(0),'isHWSink',uint8(0),'isSetup',uint8(0),'isInline',uint8(1),'isNonInline',uint8(0),'isInterrupt',uint8(0),'isChannelwise',uint8(0)),'IOBoardType','RTICAN','UnitType','MESSAGE','Identifier','RX','DialogType','MSVC','BlockSet','RTICAN','SlaveProcessor','CAN'))  RTIBlockInterface=struct('OutputPortsWidth',int32([1 1 1 1 1 1 1 1 1 1 1 1]),'OutputPortsActive',[1 1 1 1 1 1 1 1 1 1 1 1],'OutputPortsName',{{'FwdFusTrkAObjType','FwdFusTrkAMeasStatus','FwdFusTrkARelLatVel','FwdFusTrkALatPos','FwdFusTrkAConfidence','FwdFusTrkARelLongVel','FwdFusTrkALongPos','FwdFusTrkAMsgIndex','FwdFusTrkAObjectID','FwdFusTrkARollingCnt',['RX status'],['RX time']}},'OutputPortsDataType',{{'SS_DOUBLE','SS_DOUBLE','SS_DOUBLE','SS_DOUBLE','SS_DOUBLE','SS_DOUBLE','SS_DOUBLE','SS_DOUBLE','SS_DOUBLE','SS_DOUBLE','SS_DOUBLE','SS_DOUBLE'}},'OutputPortsLabel',{{'FwdFusTrkAObjType','FwdFusTrkAMeasStatus','FwdFusTrkARelLatVel','FwdFusTrkALatPos','FwdFusTrkAConfidence','FwdFusTrkARelLongVel','FwdFusTrkALongPos','FwdFusTrkAMsgIndex','FwdFusTrkAObjectID','FwdFusTrkARollingCnt','',''}},'OutputPortsLabelMode','ON','InputPortsWidth',int32(0),'InputPortsActive',0,'DialogFcn','rtican_message_interface_gui','BlockDisplay',{{'','center'}},'IconTransparency','on','ParameterTunableNames',{{}},'InitLevel',3,'BlockName',struct('Token',{{'T_Fwd_Fus_Obj_TrackA_4'}}),'SampleTime',{{-1}},'TriggerPort',{{'none'}},'EnablePort',{{'none'}})  RTIBlockParameters=struct('BoardTypeNo',{{1,'OFF',[]}},'BoardNo',{{1,'ON',[1 16]}},'ChannelNo',{{2,'ON',[1 2]}},'Parameters',{{struct('DataFileSupport',struct('DataFileSelectedMaster',1,'DataFileSelectedLocal',0,'DataFileName','c:\users\leidos\development\carmaplatform\microautobox\src\data_files\globala_fo.dbc|','DataFileDate',{{{['23-Jul-2015 14:24:26']}}},'SelectedFile',['<no file selected>']),'Options',struct('StatusSelected',1,'TimeSelected',1,'DeltaTimeSelected',0,'BytePortSelected',0,'MessageLengthSelected',0,'TriggerPort',struct('Selected',0,'TriggerType',0),'UserCoding',struct('Selected',0,'InterfaceFile','UserDecodingFile','FcnName','UserDecodeFcn','InportSelected',0,'InportWidth',1,'OutportSelected',0,'OutportWidth',1),'EnablePortSelected',0,'SignalOnPortnameSelected',1,'UseRXService',1),'Message',struct('MsgOnBlocknameSelected',1,'MsgName','T_Fwd_Fus_Obj_TrackA_4','MsgIdFormat',0,'MsgId',1812,'MsgLength',8,'NumSignals',10,'SampleTime',-1,'Signal',struct('SgnName',{'FwdFusTrkAObjType','FwdFusTrkAMeasStatus','FwdFusTrkARelLatVel','FwdFusTrkALatPos','FwdFusTrkAConfidence','FwdFusTrkARelLongVel','FwdFusTrkALongPos','FwdFusTrkAMsgIndex','FwdFusTrkAObjectID','FwdFusTrkARollingCnt'},'SgnStartBit',{0,3,5,16,27,29,40,52,56,62},'SgnLength',{3,2,11,11,2,11,12,4,6,2},'SgnType',{0,0,0,0,0,0,0,0,0,0},'ModeValue',{-1,-1,-1,-1,-1,-1,-1,-1,-1,-1},'DataType',{0,0,1,1,0,1,1,0,0,0},'ByteLayout',{2,2,2,2,2,2,2,2,2,2},'Factor',{1,1,0.125,0.125,1,0.125,0.125,1,1,1},'Offset',{0,0,0,0,0,0,0,0,0,0},'SgnComment',{{''},{''},{''},{''},{''},{''},{''},{''},{''},{''}},'SgnUnit',{'','','m/s','m','','m/s','m','','',''},'Min',{0,0,-128,-128,0,-128,-256,0,0,0},'Max',{7,3,127.875,127.875,3,127.875,255.875,15,63,3},'SLDataType',{'SS_DOUBLE','SS_DOUBLE','SS_DOUBLE','SS_DOUBLE','SS_DOUBLE','SS_DOUBLE','SS_DOUBLE','SS_DOUBLE','SS_DOUBLE','SS_DOUBLE'}),'MsgIdNumFormat',1,'MsgComment',{{''}}),'Version',1.2,'general',struct('isFromLib',0)),'OFF',[]}},'GroupId',{{struct('Group',{{'RTICAN'}},'No',2,'Behavior',{{'NAMECHANGE'}},'BlockType',{{'SINK'}},'NameChangeFlag',0),'OFF',[]}},'SFcnRTICANMessage',{{struct('MsgType','RX','SFcnPortType','Scalar','MsgName','T_Fwd_Fus_Obj_TrackA_4','MsgIdFormat','STD','MsgId',1812,'MsgLength',8,'NumSignals',10,'SampleTime',-1,'Signal',struct('SgnName',{'FwdFusTrkAObjType','FwdFusTrkAMeasStatus','FwdFusTrkARelLatVel','FwdFusTrkALatPos','FwdFusTrkAConfidence','FwdFusTrkARelLongVel','FwdFusTrkALongPos','FwdFusTrkAMsgIndex','FwdFusTrkAObjectID','FwdFusTrkARollingCnt'},'SgnStartBit',{0,3,5,16,27,29,40,52,56,62},'SgnLength',{3,2,11,11,2,11,12,4,6,2},'SgnType',{'standard','standard','standard','standard','standard','standard','standard','standard','standard','standard'},'ModeValue',{-1,-1,-1,-1,-1,-1,-1,-1,-1,-1},'DataType',{['unsigned int'],['unsigned int'],['signed int'],['signed int'],['unsigned int'],['signed int'],['signed int'],['unsigned int'],['unsigned int'],['unsigned int']},'ByteLayout',{['motorola back.'],['motorola back.'],['motorola back.'],['motorola back.'],['motorola back.'],['motorola back.'],['motorola back.'],['motorola back.'],['motorola back.'],['motorola back.']},'Factor',{1,1,0.125,0.125,1,0.125,0.125,1,1,1},'Offset',{0,0,0,0,0,0,0,0,0,0},'SLDataType',{'SS_DOUBLE','SS_DOUBLE','SS_DOUBLE','SS_DOUBLE','SS_DOUBLE','SS_DOUBLE','SS_DOUBLE','SS_DOUBLE','SS_DOUBLE','SS_DOUBLE'}),'StatusSelected','yes','TimeSelected','yes','DeltaTimeSelected','no','BytePortSelected','no','MessageLengthSelected','no','TriggerPort',struct('Selected','no','TriggerType',0),'UserCoding',struct('Selected','no','InterfaceFile','UserDecodingFile','FcnName','UserDecodeFcn','InportSelected','no','InportWidth',1,'OutportSelected','no','OutportWidth',1),'EnablePortSelected','no','UseRXService','yes','BoardType','DS1','BoardNo',1,'ControllerNo',2),'OFF',[]}},'TLCFileName',{{'rtican_rx_message','OFF',[]}})  RTISFcnParameters=struct('SFcnRTICANMessage','struct','TLCFileName','char')  RTIBlockParaDefault=struct('BoardTypeNo',4302,'BoardNo',1,'ChannelNo',1,'Parameters',struct('DataFileSupport',struct('DataFileSelectedMaster',0,'DataFileSelectedLocal',0,'DataFileName','','DataFileDate','','SelectedFile',['<no file selected>']),'Options',struct('StatusSelected',1,'TimeSelected',1,'DeltaTimeSelected',1,'BytePortSelected',0,'MessageLengthSelected',0,'TriggerPort',struct('Selected',0,'TriggerType','rising'),'UserCoding',struct('Selected',0,'InterfaceFile','UserDecodingFile','FcnName','UserDecodeFcn','InportSelected',0,'InportWidth',1,'OutportSelected',0,'OutportWidth',1),'EnablePortSelected',0,'SignalOnPortnameSelected',1,'UseRXService',0),'Message',struct('MsgOnBlocknameSelected',0,'MsgName',['RX Message'],'MsgIdFormat',0,'MsgId',100,'MsgLength',8,'NumSignals',1,'SampleTime',-1,'Signal',struct('SgnName',['RX signal'],'SgnStartBit',0,'SgnLength',8,'SgnType',0,'ModeValue',-1,'DataType',0,'SLDataType','SS_DOUBLE','ByteLayout',0,'Factor',1,'Offset',0,'Min',0,'Max',255,'SgnComment',{{}},'SgnUnit',''),'MsgIdNumFormat',0,'MsgComment',{{''}}),'Version',1.2,'general',struct('isFromLib',1)),'GroupId',struct('Group',{{'RTICAN'}},'No',1,'Behavior',{{'NAMECHANGE'}},'BlockType',{{'SINK'}},'NameChangeFlag',0),'SFcnRTICANMessage',struct('MsgType','RX','MsgName',['RX Message'],'MsgIdFormat','STD','MsgId',100,'MsgLength',8,'NumSignals',1,'SampleTime',-1,'Signal',struct('SgnName',['RX signal'],'SgnStartBit',0,'SgnLength',8,'SgnType','standard','ModeValue',-1,'DataType',['unsigned int'],'ByteLayout',['little endian'],'SLDataType','SS_DOUBLE','Factor',1,'Offset',0),'StatusSelected','yes','TimeSelected','yes','DeltaTimeSelected','yes','BytePortSelected','no','MessageLengthSelected','no','EnablePortSelected','no','UserCoding',struct('Selected','no','InterfaceFile','UserDecodingFile','FcnName','UserDecodeFcn','InportSelected','no','InportWidth',1,'OutportSelected','no','OutportWidth',1),'TriggerPort',struct('Selected','no','TriggerType','rising'),'UseRXService','no','BoardType','DS4302','BoardNo',1,'ControllerNo',1,'SFcnPortType','Scalar'),'TLCFileName','rtican_rx_message')
      settings: AttributesFormatString=Group Id: RTICAN2\n
  Vector Concatenate : Concatenate  NumInputs=4
  Object Header : Outport
  Object List : Outport  Port=2  OutDataTypeStr=Bus: FusObjectTrackA
  wires:
  T_Fwd_Fus_Obj_TrackA_1/11 -> Bus Creator/11  "Status"
  T_Fwd_Fus_Obj_TrackA_1/12 -> Bus Creator/12  "Time"
  T_Fwd_Fus_Obj_TrackA_1/1 -> Bus Creator/1  "FwdFusTrkAObjType"
  T_Fwd_Fus_Obj_TrackA_1/3 -> Bus Creator/3  "FwdFusTrkARelLatVel"
  T_Fwd_Fus_Obj_TrackA_1/2 -> Bus Creator/2  "FwdFusTrkAMeasStatus"
  T_Fwd_Fus_Obj_TrackA_1/4 -> Bus Creator/4  "FwdFusTrkALatPos"
  T_Fwd_Fus_Obj_TrackA_1/8 -> Bus Creator/8  "FwdFusTrkAMsgIndex"
  T_Fwd_Fus_Obj_TrackA_1/6 -> Bus Creator/6  "FwdFusTrkARelLongVel"
  T_Fwd_Fus_Obj_TrackA_1/5 -> Bus Creator/5  "FwdFusTrkAConfidence"
  T_Fwd_Fus_Obj_TrackA_1/7 -> Bus Creator/7  "FwdFusTrkALongPos"
  T_Fwd_Fus_Obj_TrackA_1/9 -> Bus Creator/9  "FwdFusTrkAObjectID"
  T_Fwd_Fus_Obj_TrackA_1/10 -> Bus Creator/10  "FwdFusTrkARollingCnt"
  T_Fwd_Fus_Obj_TrackA_3/1 -> Bus Creator1/1  "FwdFusTrkAObjType"
  T_Fwd_Fus_Obj_TrackA_3/9 -> Bus Creator1/9  "FwdFusTrkAObjectID"
  T_Fwd_Fus_Obj_TrackA_3/8 -> Bus Creator1/8  "FwdFusTrkAMsgIndex"
  T_Fwd_Fus_Obj_TrackA_3/4 -> Bus Creator1/4  "FwdFusTrkALatPos"
  T_Fwd_Fus_Obj_TrackA_3/5 -> Bus Creator1/5  "FwdFusTrkAConfidence"
  T_Fwd_Fus_Obj_TrackA_3/2 -> Bus Creator1/2  "FwdFusTrkAMeasStatus"
  T_Fwd_Fus_Obj_TrackA_3/10 -> Bus Creator1/10  "FwdFusTrkARollingCnt"
  T_Fwd_Fus_Obj_TrackA_3/12 -> Bus Creator1/12  "Time"
  T_Fwd_Fus_Obj_TrackA_3/3 -> Bus Creator1/3  "FwdFusTrkARelLatVel"
  T_Fwd_Fus_Obj_TrackA_3/6 -> Bus Creator1/6  "FwdFusTrkARelLongVel"
  T_Fwd_Fus_Obj_TrackA_3/7 -> Bus Creator1/7  "FwdFusTrkALongPos"
  T_Fwd_Fus_Obj_TrackA_3/11 -> Bus Creator1/11  "Status"
  T_Fwd_Fus_Obj_TrackA_2/12 -> Bus Creator2/12  "Time"
  T_Fwd_Fus_Obj_TrackA_2/1 -> Bus Creator2/1  "FwdFusTrkAObjType"
  T_Fwd_Fus_Obj_TrackA_2/5 -> Bus Creator2/5  "FwdFusTrkAConfidence"
  T_Fwd_Fus_Obj_TrackA_2/2 -> Bus Creator2/2  "FwdFusTrkAMeasStatus"
  T_Fwd_Fus_Obj_TrackA_2/4 -> Bus Creator2/4  "FwdFusTrkALatPos"
  T_Fwd_Fus_Obj_TrackA_2/11 -> Bus Creator2/11  "Status"
  T_Fwd_Fus_Obj_TrackA_2/3 -> Bus Creator2/3  "FwdFusTrkARelLatVel"
  T_Fwd_Fus_Obj_TrackA_2/7 -> Bus Creator2/7  "FwdFusTrkALongPos"
  T_Fwd_Fus_Obj_TrackA_2/8 -> Bus Creator2/8  "FwdFusTrkAMsgIndex"
  T_Fwd_Fus_Obj_TrackA_2/10 -> Bus Creator2/10  "FwdFusTrkARollingCnt"
  T_Fwd_Fus_Obj_TrackA_2/9 -> Bus Creator2/9  "FwdFusTrkAObjectID"
  T_Fwd_Fus_Obj_TrackA_2/6 -> Bus Creator2/6  "FwdFusTrkARelLongVel"
  T_Fwd_Fus_Obj_TrackA_4/12 -> Bus Creator3/12  "Time"
  T_Fwd_Fus_Obj_TrackA_4/9 -> Bus Creator3/9  "FwdFusTrkAObjectID"
  T_Fwd_Fus_Obj_TrackA_4/11 -> Bus Creator3/11  "Status"
  T_Fwd_Fus_Obj_TrackA_4/6 -> Bus Creator3/6  "FwdFusTrkARelLongVel"
  T_Fwd_Fus_Obj_TrackA_4/1 -> Bus Creator3/1  "FwdFusTrkAObjType"
  T_Fwd_Fus_Obj_TrackA_4/5 -> Bus Creator3/5  "FwdFusTrkAConfidence"
  T_Fwd_Fus_Obj_TrackA_4/8 -> Bus Creator3/8  "FwdFusTrkAMsgIndex"
  T_Fwd_Fus_Obj_TrackA_4/7 -> Bus Creator3/7  "FwdFusTrkALongPos"
  T_Fwd_Fus_Obj_TrackA_4/4 -> Bus Creator3/4  "FwdFusTrkALatPos"
  T_Fwd_Fus_Obj_TrackA_4/10 -> Bus Creator3/10  "FwdFusTrkARollingCnt"
  T_Fwd_Fus_Obj_TrackA_4/3 -> Bus Creator3/3  "FwdFusTrkARelLatVel"
  T_Fwd_Fus_Obj_TrackA_4/2 -> Bus Creator3/2  "FwdFusTrkAMeasStatus"
  Bus Creator/1 -> Vector Concatenate/1
  Bus Creator2/1 -> Vector Concatenate/2
  Bus Creator1/1 -> Vector Concatenate/3
  Bus Creator3/1 -> Vector Concatenate/4
  T_Fwd_Fus_Obj_Header/12 -> Bus Creator4/12  "T_FusHead_LrrOK"
  T_Fwd_Fus_Obj_Header/11 -> Bus Creator4/11  "T_FusHead_LFSRROK"
  T_Fwd_Fus_Obj_Header/5 -> Bus Creator4/5  "T_FusHead_RCSRROK"
  T_Fwd_Fus_Obj_Header/8 -> Bus Creator4/8  "T_FusHeadTimStmpV"
  T_Fwd_Fus_Obj_Header/7 -> Bus Creator4/7  "T_FusHeadTimStmp"
  T_Fwd_Fus_Obj_Header/9 -> Bus Creator4/9  "T_FusHead_MapDataOK"
  T_Fwd_Fus_Obj_Header/15 -> Bus Creator4/15  "T_FusHeadRollingCount"
  T_Fwd_Fus_Obj_Header/13 -> Bus Creator4/13  "T_FusHedNmValTargts"
  T_Fwd_Fus_Obj_Header/14 -> Bus Creator4/14  "T_FusHeadFuncState"
  T_Fwd_Fus_Obj_Header/1 -> Bus Creator4/1  "RoadTypeInfo"
  T_Fwd_Fus_Obj_Header/17 -> Bus Creator4/17  "Time"
  T_Fwd_Fus_Obj_Header/16 -> Bus Creator4/16  "Status"
  T_Fwd_Fus_Obj_Header/10 -> Bus Creator4/10  "T_FusHead_VIsOK"
  T_Fwd_Fus_Obj_Header/4 -> Bus Creator4/4  "T_FusHead_RFSRROK"
  T_Fwd_Fus_Obj_Header/3 -> Bus Creator4/3  "T_FusHed_ObjClstrCurv"
  T_Fwd_Fus_Obj_Header/6 -> Bus Creator4/6  "T_FusHead_LCSRROK"
  T_Fwd_Fus_Obj_Header/2 -> Bus Creator4/2  "T_FusHdObjClstTanHdng"
  Bus Creator4/1 -> Object Header/1
  Vector Concatenate/1 -> Object List/1
